simulink model "zynqRadioHWSWQPSKAD9361AD9364SL_UDP_interface"  (R2016a)
settings: Solver=FixedStepDiscrete  SolverMode=SingleTasking  StartTime=0.0  StopTime=inf  RelTol=1e-3
PreLoadFcn:
  | % Ensure SDR libraries are added to path
  | tempradiodev_ = sdrdev('ZC706 and FMCOMMS2/3/4');
  | tempradiodev_.setupSession();
  | clear tempradiodev_; % clean up
  | 
  | sdrzQPSKTxFPGA_params = zynqRadioQPSKTxFPGAAD9361AD9364SL_init;
  | sdrzQPSKrxFPGA = zynqRadioQPSKRxFPGAAD9361AD9364SL_init;
  | 
  | % ARM Tx message
  | txtstr = '*Zynq HW/SW Co-design*';
  | 
  | % Length of data set for transmit
  | DataFrameLength = 10000;
InitFcn:
  | sdrzQPSKTxFPGA_params = zynqRadioQPSKTxFPGAAD9361AD9364SL_init;
  | sdrzQPSKrxFPGA = zynqRadioQPSKRxFPGAAD9361AD9364SL_init;
  | 
  | if (numel(txtstr) > 24)
  |   error('txtstr message must be less than 24 characters');
  | end;
undefined symbols (not defined in the file or in its folder): AXI4, F, Lite, msglen, sdr
libraries: commsequence2 x2, dspsigops x2, commrandsrc2 x1, commutil2 x1, axiinterfacelib x1, zynqlib x1
CloseFcn:
  | clear sdrzQPSKrxFPGA txtstr sdrzQPSKTxFPGA_params DataFrameLength;
settings Model: DataTypeOverride=Off  SimulationMode=external  Creator=The MathWorks, Inc.  LastModifiedBy=The MathWorks, Inc.
settings SolverCC: PositivePriorityOrder=on
settings DataIOCC: LimitDataPoints=on  SaveOutput=off  SaveTime=off
settings OptimizationCC: BlockReduction=off  ConditionallyExecuteInputs=off  OptimizeModelRefInitCode=on  LifeSpan=Inf  MaxStackSize=64
settings DebuggingCC: AlgebraicLoopMsg=error  SingleTaskRateTransMsg=error  AllowSymbolicDim=off  StrictBusMsg=ErrorOnBusTreatedAsVector
settings HardwareCC: ProdBitPerPointer=32  ProdLargestAtomicInteger=Long  ProdLargestAtomicFloat=Double  ProdWordSize=32  ProdLongLongMode=on  ProdHWDeviceType=ARM Compatible->ARM Cortex
settings ModelReferenceCC: PropagateSignalLabelsOutOfModel=off
settings RTWCC: SystemTargetFile=ert.tlc  HardwareBoard=Xilinx Zynq Based Radio Board Target  TemplateMakefile=ert_default_tmf  GenerateReport=on  Toolchain=Xilinx Software Development Kit (SDK)  BuildConfiguration=Faster Runs  IncludeHyperlinkInReport=on  LaunchReport=on  GenerateTraceInfo=on  GenerateTraceReport=on  GenerateTraceReportSl=on  GenerateTraceReportSf=on  GenerateTraceReportEml=on
settings CodeAppCC: ForceParamTrailComments=on  IgnoreCustomStorageClasses=off  OperatorAnnotations=on  SimulinkDataObjDesc=on  SFDataObjDesc=on  MATLABFcnDesc=on  InsertBlockDesc=on  MATLABSourceComments=on
settings ERTTargetCC: SupportVariableSizeSignals=on
settings ConfigurationSet: Description=SimMechanics 2G

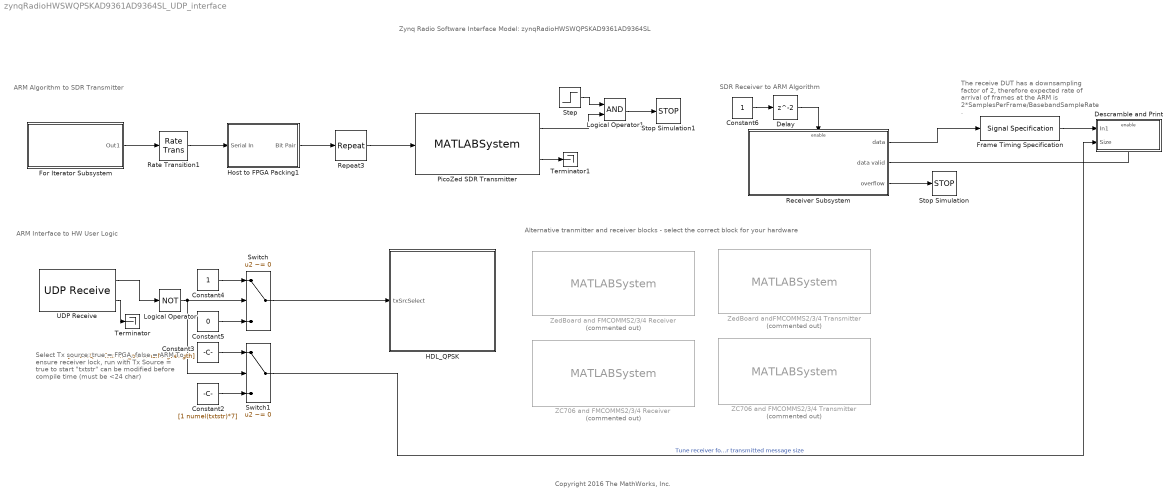
== system zynqRadioHWSWQPSKAD9361AD9364SL_UDP_interface ==
  note: Alternative tranmitter and receiver blocks - select the correct block for your hardware
  note: SDR Receiver to ARM Algorithm
  note: ARM Algorithm to SDR Transmitter
  note: ARM Interface to HW User Logic
  note: Select Tx source:
      | true = FPGA, false = ARM
      |
      | To ensure receiver lock, run with Tx
      | Source = true to start
      |
      | "txtstr" can be modified before
      | compile time (must be <24 char)
  note: Copyright 2016 The MathWorks, Inc.
  note: The receive DUT has a downsampling factor of 2, therefore expected rate of arrival of frames at the ARM is 2*SamplesPerFrame/BasebandSampleRate .
  note: Zynq Radio Software Interface Model: zynqRadioHWSWQPSKAD9361AD9364SL
  Constant2 : Constant  Value=[1 numel(txtstr)*7]  SampleTime=-1
  Constant3 : Constant  Value=[1 sdrzQPSKTxFPGA_params.MsgLength]  SampleTime=-1
  Constant4 : Constant  OutDataTypeStr=boolean  SampleTime=-1
  Constant5 : Constant  Value=0  OutDataTypeStr=boolean  SampleTime=-1
  Constant6 : Constant  SampleTime=2*(DataFrameLength/2)/sdrzQPSKrxFPGA.Fs
  Delay : Delay
  Descramble and Print : Subsystem  TreatAsAtomicUnit=on
  For Iterator Subsystem : Subsystem  TreatAsAtomicUnit=on
  Frame Timing Specification : SignalSpecification  SampleTime=2*(DataFrameLength/2)/sdrzQPSKrxFPGA.Fs
  HDL_QPSK : Subsystem  TreatAsAtomicUnit=on  mask(AXI4-Lite/AXI4 Interface){}
      mask help:
      | This is an automatically generated subsystem block.
      | This contains the AXI interface blocks that communicate with the HDL_QPSK_ip IPCore generated from zynqRadioHWSWQPSKAD9361AD9364SL/HDL_QPSK subsystem.
      mask Display: disp(sprintf('Xilinx Zynq \nAXI Interface'));
  Host to FPGA Packing1 : Subsystem
  Logical Operator : Logic  Operator=NOT  AllPortsSameDT=off  OutDataTypeStr=boolean
  Logical Operator1 : Logic  AllPortsSameDT=off  OutDataTypeStr=boolean
  PicoZed SDR Transmitter : MATLABSystem  Priority=0  InitFcn=sdr.internal.registerBlocks(gcb, 'xpicozedsdr');  System=comm.internal.SDRTxPicoZedSDRSL  IPAddress=192.168.3.2  CenterFrequencySource=Dialog  CenterFrequency=2400000000  GainSource=Dialog  Gain=-10  ChannelMapping=1  BasebandSampleRate=sdrzQPSKrxFPGA.Fs  EnableBurstMode=off  NumFramesInBurst=20  DMATimeoutValue=200e-6  EnableTxPrimingMode=on  blockMode=Codegen  LostSamplesOutputPort=on  OverflowOutputPort=off  DataSourceSelect=Host  DDSFrequency=[ 1000000, 1000000; 1000000, 1000000 ]  DDSPhase=[ 0, 0; 0, 0 ]  DDSScale=[ 250000, 250000; 250000, 250000 ]  BypassUserLogic=off  ShowAdvancedProperties=on  ShowInternalProperties=off  subDeviceList=zynqTransmitter  sdrExecutionMode=HW  dataUDPPort=-1  ctrlUDPPort=-1  FIRCoefficientSize=[ 128; 128 ]  FIRCoefficients=[ 111, -87, 147, -127, -18, -286, -312, -555, -601, -722, -642, -555, -303, -66, 221, 393, 488, 403, 219, -74, -343, -550, -582, -450, -146, 221, 569, 759, 735, 463, 20, -487, -885, -1048, -883, -418, 243, 897, 1340, 1394, 1002, 228, -715, -1549, -1980, -1819, -1028, 217, 1583, 2635, 2980, 2377, 853, -1275, -3435, -4926, -5080, -3454, 40, 5065, 10903, 16581, 21085, 23573, 23573, 21085, 16581, 10903, 5065, 40, -3454, -5080, -4926, -3435, -1275, 853, 2377, 2980, 2635, 1583, 217, -1028, -1819, -1980, -1549, -715, 228, 1002, 1394, 1340, 897, 243, -418, -883, -1048, -885, -487, 20, 463, 735, 759, 569, 221, -146, -450, -582, -550, -343, -74, 219, 403, 488, 393, 221, -66, -303, -555, -642, -722, -601, -555, -312, -286, -18, -127, 147, -87, 111; 382, -200, 711, -41, 645, 36, 346, -194, -119, -543, -472, -646, -404, -312, 45, 197, 413, 346, 241, -93, -373, -680, -755, -689, -356, 51, 515, 795, 870, 609, 136, -488, -1009, -1303, -1191, -712, 69, 885, 1516, 1692, 1336, 468, -662, -1740, -2378, -2329, -1494, -55, 1620, 2995, 3584, 3045, 1368, -1121, -3755, -5708, -6156, -4542, -710, 4969, 11669, 18243, 23486, 26391, 26391, 23486, 18243, 11669, 4969, -710, -4542, -6156, -5708, -3755, -1121, 1368, 3045, 3584, 2995, 1620, -55, -1494, -2329, -2378, -1740, -662, 468, 1336, 1692, 1516, 885, 69, -712, -1191, -1303, -1009, -488, 136, 609, 870, 795, 515, 51, -356, -689, -755, -680, -373, -93, 241, 346, 413, 197, 45, -312, -404, -646, -472, -543, -119, -194, 346, 36, 645, -41, 711, -200, 382 ]  FIRGain=[ 0; -12 ]  FIRDecimInterpFactor=[ 4; 4 ]  AnalogFilterCutoff=[ 2560000; 2560000 ]  FilterPathRates=[ 737280000, 184320000, 61440000, 30720000, 15360000, 3840000; 737280000, 184320000, 61440000, 30720000, 15360000, 3840000 ]  FilterDesignTypeForTx=DefaultFilter  FilterDesignTypeForRx=DefaultFilterFromOther  SimulateUsing=Interpreted execution
      mask Type: comm.internal.SDRTxPicoZedSDRSL
      mask Display:
      | disp(['PicoZed SDR' char(10) 'ARM-FPGA Interface']);
      | port_label('input',1,'data');
      | port_label('output',1,'underflow');
      | port_label('output',2,'overflow');
  Rate Transition1 : RateTransition  OutPortSampleTime=sdrzQPSKTxFPGA_params.FrameTime*(DataFrameLength/(sdrzQPSKTxFPGA_params.DataLength + 2*sdrzQPSKTxFPGA_params.BarkerLength))
  Receiver Subsystem : Subsystem
  Repeat3 : dspsigops/Repeat  N=4  InputProcessing=Columns as channels (frame based)  RateOptions=Allow multirate processing  ic=0  mode=Unused parameter value
  Step : Step  Time=10*DataFrameLength/sdrzQPSKrxFPGA.Fs  SampleTime=DataFrameLength/sdrzQPSKrxFPGA.Fs
  Stop Simulation : Stop
  Stop Simulation1 : Stop
  Switch : Switch  Criteria=u2 ~= 0
  Switch1 : Switch  Criteria=u2 ~= 0
  Terminator : Terminator
  Terminator1 : Terminator
  UDP Receive : zynqlib/UDP Receive  localURL='0.0.0.0'  localPort=25000  remoteURL='0.0.0.0'  remotePort=-1  recvBufferSize=8192  dims=1  signalDatatype=boolean  isVarSize=off  showBlockingTime=on  blockingTime=0  sampletime=2*(DataFrameLength/2)/sdrzQPSKrxFPGA.Fs  blockPlatform=ZYNQ
  ZC706 and FMCOMMS2/3/4 Receiver : MATLABSystem  Priority=0  Commented=on  InitFcn=sdr.internal.registerBlocks(gcb, 'xzc706afmc3');  System=comm.internal.SDRRxZC706FMC234SL  IPAddress=192.168.3.2  CenterFrequencySource=Dialog  CenterFrequency=2400000000  GainSource=AGC Slow Attack  Gain=1  ChannelMapping=1  BasebandSampleRate=sdrzQPSKrxFPGA.Fs  EnableBurstMode=off  NumFramesInBurst=20  OutputDataType=int16  SamplesPerFrame=DataFrameLength/2  LostSamplesOutputPort=on  RSSIOutputPort=off  DMATimeoutValue=200e-6  blockMode=Codegen  EnableQuadratureTracking=on  EnableRFDCTracking=on  EnableBasebandDCTracking=on  BypassUserLogic=off  ShowAdvancedProperties=on  ShowInternalProperties=off  subDeviceList=zynqReceiver  sdrExecutionMode=HW  dataUDPPort=-1  ctrlUDPPort=-1  SourceSelect=RF data  SourceConfiguration1=1023  FIRCoefficientSize=[128;128]  FIRCoefficients=[55 -54 42 -126 -123 -317 -399 -581 -646 -711 -634 -507 -263 -10 255 424 492 401 201 -84 -352 -540 -566 -423 -126 234 562 738 701 429 -5 -490 -866 -1007 -834 -372 266 891 1301 1334 936 178 -733 -1524 -1917 -1731 -944 274 1590 2585 2881 2255 741 -1344 -3435 -4850 -4942 -3285 197 5169 10923 16509 20932 23375 23375 20932 16509 10923 5169 197 -3285 -4942 -4850 -3435 -1344 741 2255 2881 2585 1590 274 -944 -1731 -1917 -1524 -733 178 936 1334 1301 891 266 -372 -834 -1007 -866 -490 -5 429 701 738 562 234 -126 -423 -566 -540 -352 -84 201 401 492 424 255 -10 -263 -507 -634 -711 -646 -581 -399 -317 -123 -126 42 -54 55;190 -88 329 -40 239 -99 -24 -349 -377 -611 -573 -604 -395 -229 66 239 394 350 227 -46 -300 -534 -593 -506 -221 137 512 737 765 526 103 -420 -852 -1069 -947 -512 156 841 1341 1450 1100 333 -638 -1531 -2028 -1922 -1152 115 1544 2677 3099 2535 997 -1205 -3479 -5095 -5345 -3750 -199 4965 11002 16895 21580 24172 24172 21580 16895 11002 4965 -199 -3750 -5345 -5095 -3479 -1205 997 2535 3099 2677 1544 115 -1152 -1922 -2028 -1531 -638 333 1100 1450 1341 841 156 -512 -947 -1069 -852 -420 103 526 765 737 512 137 -221 -506 -593 -534 -300 -46 227 350 394 239 66 -229 -395 -604 -573 -611 -377 -349 -24 -99 239 -40 329 -88 190]  FIRGain=[0;-12]  FIRDecimInterpFactor=[4;4]  AnalogFilterCutoff=[3152524;3161715]  FilterPathRates=[983040000 122880000 61440000 30720000 15360000 3840000;983040000 122880000 61440000 30720000 15360000 3840000]  FilterDesignTypeForTx=DefaultFilterFromOther  FilterDesignTypeForRx=DefaultFilter  BISTLoopbackConfig=No Loopback  BISTPRBSMode=PRBS Disable  BISTToneMode=Tone Disable  BISTToneFrequency=F/32  BISTToneLevel=-6  BISTChannelMask=0  DataIsComplex=on  SimulateUsing=Interpreted execution
      mask Type: comm.internal.SDRRxZC706FMC234SL
      mask Display:
      | disp(['ZC706 and FMCOMMS2/3/4' char(10) 'ARM-FPGA Interface']);
      | port_label('output',1,'data');
      | port_label('output',2,'data valid');
      | port_label('output',3,'overflow');
  ZC706 and FMCOMMS2/3/4 Transmitter : MATLABSystem  Commented=on  InitFcn=sdr.internal.registerBlocks(gcb, 'xzc706afmc3');  System=comm.internal.SDRTxZC706FMC234SL  IPAddress=192.168.3.2  CenterFrequencySource=Dialog  CenterFrequency=2400000000  GainSource=Dialog  Gain=-10  ChannelMapping=1  BasebandSampleRate=sdrzQPSKrxFPGA.Fs  EnableBurstMode=off  NumFramesInBurst=20  DMATimeoutValue=200e-6  EnableTxPrimingMode=on  blockMode=Codegen  LostSamplesOutputPort=on  OverflowOutputPort=off  DataSourceSelect=Host  DDSFrequency=1000000*ones([2 2])  DDSPhase=[0 0;0 0]  DDSScale=250000*ones([2 2])  BypassUserLogic=off  ShowAdvancedProperties=on  ShowInternalProperties=off  subDeviceList=zynqTransmitter  sdrExecutionMode=HW  dataUDPPort=-1  ctrlUDPPort=-1  FIRCoefficientSize=[128;128]  FIRCoefficients=[55 -54 42 -126 -123 -317 -399 -581 -646 -711 -634 -507 -263 -10 255 424 492 401 201 -84 -352 -540 -566 -423 -126 234 562 738 701 429 -5 -490 -866 -1007 -834 -372 266 891 1301 1334 936 178 -733 -1524 -1917 -1731 -944 274 1590 2585 2881 2255 741 -1344 -3435 -4850 -4942 -3285 197 5169 10923 16509 20932 23375 23375 20932 16509 10923 5169 197 -3285 -4942 -4850 -3435 -1344 741 2255 2881 2585 1590 274 -944 -1731 -1917 -1524 -733 178 936 1334 1301 891 266 -372 -834 -1007 -866 -490 -5 429 701 738 562 234 -126 -423 -566 -540 -352 -84 201 401 492 424 255 -10 -263 -507 -634 -711 -646 -581 -399 -317 -123 -126 42 -54 55;190 -88 329 -40 239 -99 -24 -349 -377 -611 -573 -604 -395 -229 66 239 394 350 227 -46 -300 -534 -593 -506 -221 137 512 737 765 526 103 -420 -852 -1069 -947 -512 156 841 1341 1450 1100 333 -638 -1531 -2028 -1922 -1152 115 1544 2677 3099 2535 997 -1205 -3479 -5095 -5345 -3750 -199 4965 11002 16895 21580 24172 24172 21580 16895 11002 4965 -199 -3750 -5345 -5095 -3479 -1205 997 2535 3099 2677 1544 115 -1152 -1922 -2028 -1531 -638 333 1100 1450 1341 841 156 -512 -947 -1069 -852 -420 103 526 765 737 512 137 -221 -506 -593 -534 -300 -46 227 350 394 239 66 -229 -395 -604 -573 -611 -377 -349 -24 -99 239 -40 329 -88 190]  FIRGain=[0;-12]  FIRDecimInterpFactor=[4;4]  AnalogFilterCutoff=[3152524;3161715]  FilterPathRates=[983040000 122880000 61440000 30720000 15360000 3840000;983040000 122880000 61440000 30720000 15360000 3840000]  FilterDesignTypeForTx=DefaultFilter  FilterDesignTypeForRx=DefaultFilterFromOther  SimulateUsing=Interpreted execution
      mask Type: comm.internal.SDRTxZC706FMC234SL
      mask Display:
      | disp(['ZC706 and FMCOMMS2/3/4' char(10) 'ARM-FPGA Interface']);
      | port_label('input',1,'data');
      | port_label('output',1,'underflow');
      | port_label('output',2,'overflow');
  ZedBoard and FMCOMMS2/3/4 Receiver : MATLABSystem  Priority=0  Commented=on  InitFcn=sdr.internal.registerBlocks(gcb, 'xzedboardafmc3');  System=comm.internal.SDRRxZedBoardFMC234SL  IPAddress=192.168.3.2  CenterFrequencySource=Dialog  CenterFrequency=2400000000  GainSource=AGC Slow Attack  Gain=1  ChannelMapping=1  BasebandSampleRate=sdrzQPSKrxFPGA.Fs  EnableBurstMode=off  NumFramesInBurst=20  OutputDataType=int16  SamplesPerFrame=DataFrameLength/2  LostSamplesOutputPort=on  RSSIOutputPort=off  DMATimeoutValue=200e-6  blockMode=Codegen  EnableQuadratureTracking=on  EnableRFDCTracking=on  EnableBasebandDCTracking=on  BypassUserLogic=off  ShowAdvancedProperties=on  ShowInternalProperties=off  subDeviceList=zynqReceiver  sdrExecutionMode=HW  dataUDPPort=-1  ctrlUDPPort=-1  SourceSelect=RF data  SourceConfiguration1=1023  FIRCoefficientSize=[ 128; 128 ]  FIRCoefficients=[ 111, -87, 147, -127, -18, -286, -312, -555, -601, -722, -642, -555, -303, -66, 221, 393, 488, 403, 219, -74, -343, -550, -582, -450, -146, 221, 569, 759, 735, 463, 20, -487, -885, -1048, -883, -418, 243, 897, 1340, 1394, 1002, 228, -715, -1549, -1980, -1819, -1028, 217, 1583, 2635, 2980, 2377, 853, -1275, -3435, -4926, -5080, -3454, 40, 5065, 10903, 16581, 21085, 23573, 23573, 21085, 16581, 10903, 5065, 40, -3454, -5080, -4926, -3435, -1275, 853, 2377, 2980, 2635, 1583, 217, -1028, -1819, -1980, -1549, -715, 228, 1002, 1394, 1340, 897, 243, -418, -883, -1048, -885, -487, 20, 463, 735, 759, 569, 221, -146, -450, -582, -550, -343, -74, 219, 403, 488, 393, 221, -66, -303, -555, -642, -722, -601, -555, -312, -286, -18, -127, 147, -87, 111; 382, -200, 711, -41, 645, 36, 346, -194, -119, -543, -472, -646, -404, -312, 45, 197, 413, 346, 241, -93, -373, -680, -755, -689, -356, 51, 515, 795, 870, 609, 136, -488, -1009, -1303, -1191, -712, 69, 885, 1516, 1692, 1336, 468, -662, -1740, -2378, -2329, -1494, -55, 1620, 2995, 3584, 3045, 1368, -1121, -3755, -5708, -6156, -4542, -710, 4969, 11669, 18243, 23486, 26391, 26391, 23486, 18243, 11669, 4969, -710, -4542, -6156, -5708, -3755, -1121, 1368, 3045, 3584, 2995, 1620, -55, -1494, -2329, -2378, -1740, -662, 468, 1336, 1692, 1516, 885, 69, -712, -1191, -1303, -1009, -488, 136, 609, 870, 795, 515, 51, -356, -689, -755, -680, -373, -93, 241, 346, 413, 197, 45, -312, -404, -646, -472, -543, -119, -194, 346, 36, 645, -41, 711, -200, 382 ]  FIRGain=[ 0; -12 ]  FIRDecimInterpFactor=[ 4; 4 ]  AnalogFilterCutoff=[ 2560000; 2560000 ]  FilterPathRates=[ 737280000, 184320000, 61440000, 30720000, 15360000, 3840000; 737280000, 184320000, 61440000, 30720000, 15360000, 3840000 ]  FilterDesignTypeForTx=DefaultFilterFromOther  FilterDesignTypeForRx=DefaultFilter  BISTLoopbackConfig=No Loopback  BISTPRBSMode=PRBS Disable  BISTToneMode=Tone Disable  BISTToneFrequency=F/32  BISTToneLevel=-6  BISTChannelMask=0  DataIsComplex=on  SimulateUsing=Interpreted execution
      mask Type: comm.internal.SDRRxZedBoardFMC234SL
      mask Display:
      | disp(['ZedBoard and FMCOMMS2/3/4' char(10) 'ARM-FPGA Interface']);
      | port_label('output',1,'data');
      | port_label('output',2,'data valid');
      | port_label('output',3,'overflow');
  ZedBoard andFMCOMMS2/3/4 Transmitter : MATLABSystem  Commented=on  InitFcn=sdr.internal.registerBlocks(gcb, 'xzedboardafmc3');  System=comm.internal.SDRTxZedBoardFMC234SL  IPAddress=192.168.3.2  CenterFrequencySource=Dialog  CenterFrequency=2400000000  GainSource=Dialog  Gain=-10  ChannelMapping=1  BasebandSampleRate=sdrzQPSKrxFPGA.Fs  EnableBurstMode=off  NumFramesInBurst=20  DMATimeoutValue=200e-6  EnableTxPrimingMode=on  blockMode=Codegen  LostSamplesOutputPort=on  OverflowOutputPort=off  DataSourceSelect=Host  DDSFrequency=[ 1000000, 1000000; 1000000, 1000000 ]  DDSPhase=[ 0, 0; 0, 0 ]  DDSScale=[ 250000, 250000; 250000, 250000 ]  BypassUserLogic=off  ShowAdvancedProperties=on  ShowInternalProperties=off  subDeviceList=zynqTransmitter  sdrExecutionMode=HW  dataUDPPort=-1  ctrlUDPPort=-1  FIRCoefficientSize=[ 128; 128 ]  FIRCoefficients=[ 111, -87, 147, -127, -18, -286, -312, -555, -601, -722, -642, -555, -303, -66, 221, 393, 488, 403, 219, -74, -343, -550, -582, -450, -146, 221, 569, 759, 735, 463, 20, -487, -885, -1048, -883, -418, 243, 897, 1340, 1394, 1002, 228, -715, -1549, -1980, -1819, -1028, 217, 1583, 2635, 2980, 2377, 853, -1275, -3435, -4926, -5080, -3454, 40, 5065, 10903, 16581, 21085, 23573, 23573, 21085, 16581, 10903, 5065, 40, -3454, -5080, -4926, -3435, -1275, 853, 2377, 2980, 2635, 1583, 217, -1028, -1819, -1980, -1549, -715, 228, 1002, 1394, 1340, 897, 243, -418, -883, -1048, -885, -487, 20, 463, 735, 759, 569, 221, -146, -450, -582, -550, -343, -74, 219, 403, 488, 393, 221, -66, -303, -555, -642, -722, -601, -555, -312, -286, -18, -127, 147, -87, 111; 382, -200, 711, -41, 645, 36, 346, -194, -119, -543, -472, -646, -404, -312, 45, 197, 413, 346, 241, -93, -373, -680, -755, -689, -356, 51, 515, 795, 870, 609, 136, -488, -1009, -1303, -1191, -712, 69, 885, 1516, 1692, 1336, 468, -662, -1740, -2378, -2329, -1494, -55, 1620, 2995, 3584, 3045, 1368, -1121, -3755, -5708, -6156, -4542, -710, 4969, 11669, 18243, 23486, 26391, 26391, 23486, 18243, 11669, 4969, -710, -4542, -6156, -5708, -3755, -1121, 1368, 3045, 3584, 2995, 1620, -55, -1494, -2329, -2378, -1740, -662, 468, 1336, 1692, 1516, 885, 69, -712, -1191, -1303, -1009, -488, 136, 609, 870, 795, 515, 51, -356, -689, -755, -680, -373, -93, 241, 346, 413, 197, 45, -312, -404, -646, -472, -543, -119, -194, 346, 36, 645, -41, 711, -200, 382 ]  FIRGain=[ 0; -12 ]  FIRDecimInterpFactor=[ 4; 4 ]  AnalogFilterCutoff=[ 2560000; 2560000 ]  FilterPathRates=[ 737280000, 184320000, 61440000, 30720000, 15360000, 3840000; 737280000, 184320000, 61440000, 30720000, 15360000, 3840000 ]  FilterDesignTypeForTx=DefaultFilter  FilterDesignTypeForRx=DefaultFilterFromOther  SimulateUsing=Interpreted execution
      mask Type: comm.internal.SDRTxZedBoardFMC234SL
      mask Display:
      | disp(['ZedBoard and FMCOMMS2/3/4' char(10) 'ARM-FPGA Interface']);
      | port_label('input',1,'data');
      | port_label('output',1,'underflow');
      | port_label('output',2,'overflow');
  wires:
  Repeat3/1 -> PicoZed SDR Transmitter/1
  Frame Timing Specification/1 -> Descramble and Print/1(In1)
  Switch/1 -> HDL_QPSK/1(txSrcSelect)
  Constant4/1 -> Switch/1
  Constant5/1 -> Switch/3
  Constant2/1 -> Switch1/3
  Constant3/1 -> Switch1/1
  Switch1/1 -> Descramble and Print/2(Size)  "Tune receiver for transmitted message size"
  PicoZed SDR Transmitter/2 -> Terminator1/1
  For Iterator Subsystem/1(Out1) -> Rate Transition1/1
  Host to FPGA Packing1/1(Bit Pair) -> Repeat3/1
  Rate Transition1/1 -> Host to FPGA Packing1/1(Serial In)
  Receiver Subsystem/1(data) -> Frame Timing Specification/1
  Receiver Subsystem/2(data valid) -> Descramble and Print/Enable
  Receiver Subsystem/3(overflow) -> Stop Simulation/1
  Constant6/1 -> Delay/1
  Delay/1 -> Receiver Subsystem/Enable
  Logical Operator/1 -> Switch1/2, Switch/2
  UDP Receive/1 -> Logical Operator/1
  Step/1 -> Logical Operator1/1
  PicoZed SDR Transmitter/1 -> Logical Operator1/2
  UDP Receive/2 -> Terminator/1
  Logical Operator1/1 -> Stop Simulation1/1

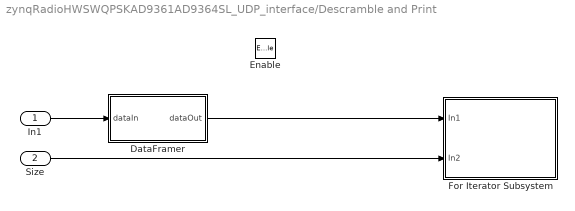
== system zynqRadioHWSWQPSKAD9361AD9364SL_UDP_interface/Descramble and Print ==
  In1 : Inport
  Size : Inport  Port=2
  Enable : EnablePort  PropagateVarSize=During execution
  DataFramer : MATLAB Function  TreatAsAtomicUnit=on
  For Iterator Subsystem : Subsystem  TreatAsAtomicUnit=on
  wires:
  In1/1 -> DataFramer/1(dataIn)
  DataFramer/1(dataOut) -> For Iterator Subsystem/1(In1)
  Size/1 -> For Iterator Subsystem/2(In2)

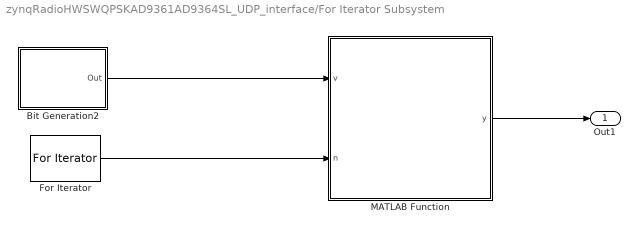
== system zynqRadioHWSWQPSKAD9361AD9364SL_UDP_interface/For Iterator Subsystem ==
  Bit Generation2 : Subsystem
      mask Display: disp('Bits Generation')
  For Iterator : ForIterator  IterationLimit=(DataFrameLength/(sdrzQPSKTxFPGA_params.DataLength + 2*sdrzQPSKTxFPGA_params.BarkerLength))-1  IndexMode=Zero-based
  MATLAB Function : MATLAB Function  TreatAsAtomicUnit=on
  Out1 : Outport
  wires:
  MATLAB Function/1(y) -> Out1/1
  For Iterator/1 -> MATLAB Function/2(n)
  Bit Generation2/1(Out) -> MATLAB Function/1(v)

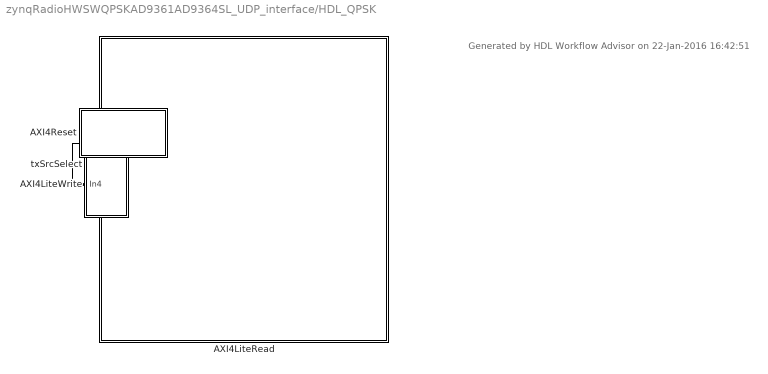
== system zynqRadioHWSWQPSKAD9361AD9364SL_UDP_interface/HDL_QPSK ==
  note: Generated by HDL Workflow Advisor on 22-Jan-2016 16:42:51
  txSrcSelect : Inport
  AXI4LiteRead : Subsystem  Priority=10
  AXI4LiteWrite : Subsystem  Priority=1
  AXI4Reset : Subsystem  mask(System Initialize){ShowInLibBrowser=0}
      mask prompts: ShowInLibBrowser "Simulink:masks:CustCodeMaskParam1_MP"
      settings: CopyFcn=cccopyfcn(gcb)  OpenFcn=ccopenfcn('System Initialize Function')
      mask Help: eval('feval(''rtwprivate'',''rtwhelpview'',''rtw_sys_initialize_block'')');
      mask Display: disp('System\nInitialize');
  wires:
  txSrcSelect/1 -> AXI4LiteWrite/1(In4)

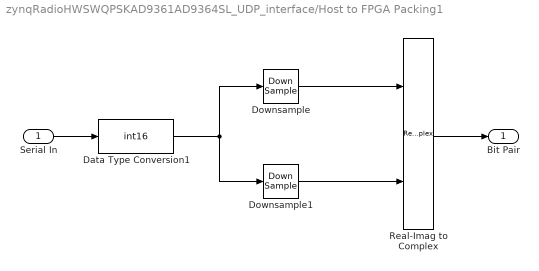
== system zynqRadioHWSWQPSKAD9361AD9364SL_UDP_interface/Host to FPGA Packing1 ==
  Serial In : Inport
  Data Type Conversion1 : DataTypeConversion  OutDataTypeStr=int16
  Downsample : DownSample  RateOptions=Allow multirate processing
  Downsample1 : DownSample  phase=1  RateOptions=Allow multirate processing
  Real-Imag to Complex : RealImagToComplex
  Bit Pair : Outport
  wires:
  Downsample/1 -> Real-Imag to Complex/1
  Serial In/1 -> Data Type Conversion1/1
  Data Type Conversion1/1 -> Downsample1/1, Downsample/1
  Downsample1/1 -> Real-Imag to Complex/2
  Real-Imag to Complex/1 -> Bit Pair/1

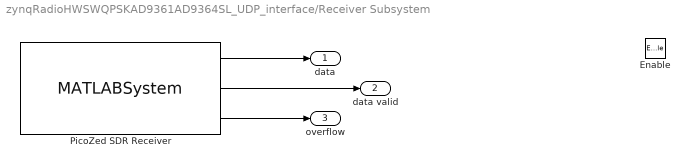
== system zynqRadioHWSWQPSKAD9361AD9364SL_UDP_interface/Receiver Subsystem ==
  Enable : EnablePort
  PicoZed SDR Receiver : MATLABSystem  InitFcn=sdr.internal.registerBlocks(gcb, 'xpicozedsdr');  System=comm.internal.SDRRxPicoZedSDRSL  IPAddress=192.168.3.2  CenterFrequencySource=Dialog  CenterFrequency=2400000000  GainSource=AGC Fast Attack  Gain=1  ChannelMapping=1  BasebandSampleRate=sdrzQPSKrxFPGA.Fs  EnableBurstMode=off  NumFramesInBurst=20  OutputDataType=int16  SamplesPerFrame=DataFrameLength/2  LostSamplesOutputPort=on  RSSIOutputPort=off  DMATimeoutValue=200e-6  blockMode=Codegen  EnableQuadratureTracking=on  EnableRFDCTracking=on  EnableBasebandDCTracking=on  BypassUserLogic=off  ShowAdvancedProperties=on  ShowInternalProperties=off  subDeviceList=zynqReceiver  sdrExecutionMode=HW  dataUDPPort=-1  ctrlUDPPort=-1  SourceSelect=RF data  SourceConfiguration1=1023  FIRCoefficientSize=[ 128; 128 ]  FIRCoefficients=[ 111, -87, 147, -127, -18, -286, -312, -555, -601, -722, -642, -555, -303, -66, 221, 393, 488, 403, 219, -74, -343, -550, -582, -450, -146, 221, 569, 759, 735, 463, 20, -487, -885, -1048, -883, -418, 243, 897, 1340, 1394, 1002, 228, -715, -1549, -1980, -1819, -1028, 217, 1583, 2635, 2980, 2377, 853, -1275, -3435, -4926, -5080, -3454, 40, 5065, 10903, 16581, 21085, 23573, 23573, 21085, 16581, 10903, 5065, 40, -3454, -5080, -4926, -3435, -1275, 853, 2377, 2980, 2635, 1583, 217, -1028, -1819, -1980, -1549, -715, 228, 1002, 1394, 1340, 897, 243, -418, -883, -1048, -885, -487, 20, 463, 735, 759, 569, 221, -146, -450, -582, -550, -343, -74, 219, 403, 488, 393, 221, -66, -303, -555, -642, -722, -601, -555, -312, -286, -18, -127, 147, -87, 111; 382, -200, 711, -41, 645, 36, 346, -194, -119, -543, -472, -646, -404, -312, 45, 197, 413, 346, 241, -93, -373, -680, -755, -689, -356, 51, 515, 795, 870, 609, 136, -488, -1009, -1303, -1191, -712, 69, 885, 1516, 1692, 1336, 468, -662, -1740, -2378, -2329, -1494, -55, 1620, 2995, 3584, 3045, 1368, -1121, -3755, -5708, -6156, -4542, -710, 4969, 11669, 18243, 23486, 26391, 26391, 23486, 18243, 11669, 4969, -710, -4542, -6156, -5708, -3755, -1121, 1368, 3045, 3584, 2995, 1620, -55, -1494, -2329, -2378, -1740, -662, 468, 1336, 1692, 1516, 885, 69, -712, -1191, -1303, -1009, -488, 136, 609, 870, 795, 515, 51, -356, -689, -755, -680, -373, -93, 241, 346, 413, 197, 45, -312, -404, -646, -472, -543, -119, -194, 346, 36, 645, -41, 711, -200, 382 ]  FIRGain=[ 0; -12 ]  FIRDecimInterpFactor=[ 4; 4 ]  AnalogFilterCutoff=[ 2560000; 2560000 ]  FilterPathRates=[ 737280000, 184320000, 61440000, 30720000, 15360000, 3840000; 737280000, 184320000, 61440000, 30720000, 15360000, 3840000 ]  FilterDesignTypeForTx=DefaultFilterFromOther  FilterDesignTypeForRx=DefaultFilter  BISTLoopbackConfig=No Loopback  BISTPRBSMode=PRBS Disable  BISTToneMode=Tone Disable  BISTToneFrequency=F/32  BISTToneLevel=-6  BISTChannelMask=0  DataIsComplex=on  SimulateUsing=Interpreted execution
      mask Type: comm.internal.SDRRxPicoZedSDRSL
      mask Display:
      | disp(['PicoZed SDR' char(10) 'ARM-FPGA Interface']);
      | port_label('output',1,'data');
      | port_label('output',2,'data valid');
      | port_label('output',3,'overflow');
  data : Outport
  data valid : Outport  Port=2
  overflow : Outport  Port=3
  wires:
  PicoZed SDR Receiver/2 -> data valid/1
  PicoZed SDR Receiver/1 -> data/1
  PicoZed SDR Receiver/3 -> overflow/1

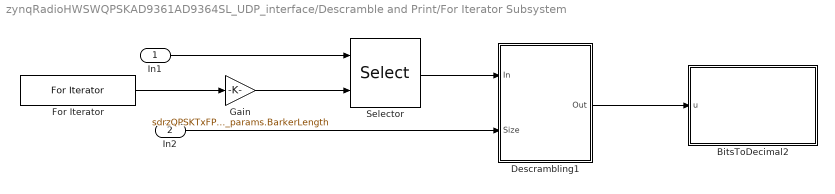
== system zynqRadioHWSWQPSKAD9361AD9364SL_UDP_interface/Descramble and Print/For Iterator Subsystem ==
  In1 : Inport
  In2 : Inport  Port=2
  BitsToDecimal2 : MATLAB Function  TreatAsAtomicUnit=on
  Descrambling1 : Subsystem
      mask Display: disp('Descrambling')
  For Iterator : ForIterator  IterationLimit=(DataFrameLength/(sdrzQPSKTxFPGA_params.DataLength + 2*sdrzQPSKTxFPGA_params.BarkerLength))-1  IndexMode=Zero-based
  Gain : Gain  Gain=sdrzQPSKTxFPGA_params.DataLength + 2*sdrzQPSKTxFPGA_params.BarkerLength  OutDataTypeStr=int32
  Selector : Selector  IndexMode=Zero-based  IndexOptions=Starting index (port)  Indices=[sdrzQPSKrxFPGA.BarkerLength*log2(sdrzQPSKrxFPGA.M)+1:sdrzQPSKrxFPGA.FrameSize*log2(sdrzQPSKrxFPGA.M)]  OutputSizes=sdrzQPSKTxFPGA_params.DataLength + 2*sdrzQPSKTxFPGA_params.BarkerLength
  wires:
  Descrambling1/1(Out) -> BitsToDecimal2/1(u)
  In2/1 -> Descrambling1/2(Size)
  In1/1 -> Selector/1
  Selector/1 -> Descrambling1/1(In)
  Gain/1 -> Selector/2
  For Iterator/1 -> Gain/1

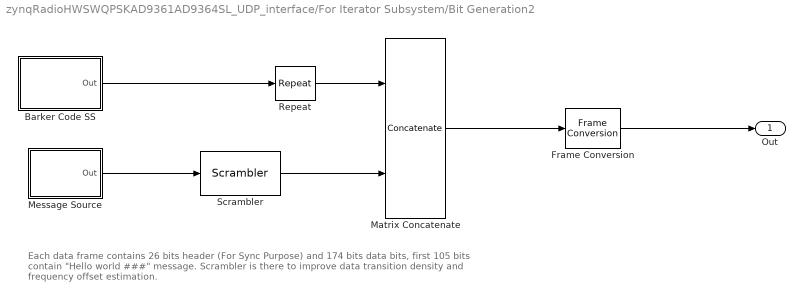
== system zynqRadioHWSWQPSKAD9361AD9364SL_UDP_interface/For Iterator Subsystem/Bit Generation2 ==
  note: Each data frame contains 26 bits header (For Sync Purpose) and 174 bits data bits,
      | first 105 bits contain "Hello world ###" message. Scrambler is there to improve data
      | transition density and frequency offset estimation.
  Barker Code SS : Subsystem
      mask Display: disp('Unipolar\nBarker Code')
  Frame Conversion : FrameConversion  InheritSamplingMode=off  OutFrame=Sample-based
  Matrix Concatenate : Concatenate  Mode=Multidimensional array
  Message Source : Subsystem
      mask Display: disp('Message\nSource')
  Repeat : dspsigops/Repeat  N=2  InputProcessing=Columns as channels (frame based)  RateOptions=Enforce single-rate processing  ic=0  mode=Unused parameter value
  Scrambler : commsequence2/Scrambler  M=2  poly=[1 1 1 0 1]  iniStaSource=Dialog Parameter  ini_sta=[0 0 0 0]  resetViaPort=off
  Out : Outport
  wires:
  Frame Conversion/1 -> Out/1
  Matrix Concatenate/1 -> Frame Conversion/1
  Barker Code SS/1(Out) -> Repeat/1
  Repeat/1 -> Matrix Concatenate/1
  Scrambler/1 -> Matrix Concatenate/2
  Message Source/1(Out) -> Scrambler/1

== system zynqRadioHWSWQPSKAD9361AD9364SL_UDP_interface/HDL_QPSK/AXI4LiteRead ==

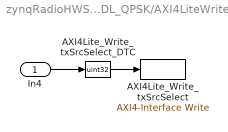
== system zynqRadioHWSWQPSKAD9361AD9364SL_UDP_interface/HDL_QPSK/AXI4LiteWrite ==
  In4 : Inport
  AXI4Lite_Write_txSrcSelect : axiinterfacelib/AXI4-Interface Write  Priority=7  AXIInterfaceType=AXI4-Lite  DeviceName=/dev/mwipcore1  RegisterOffset=hex2dec('100')  blockPlatform=ZYNQ  SimulateUsing=Interpreted execution
  AXI4Lite_Write_txSrcSelect_DTC : DataTypeConversion  OutDataTypeStr=uint32  ConvertRealWorld=Stored Integer (SI)
  wires:
  In4/1 -> AXI4Lite_Write_txSrcSelect_DTC/1
  AXI4Lite_Write_txSrcSelect_DTC/1 -> AXI4Lite_Write_txSrcSelect/1

== system zynqRadioHWSWQPSKAD9361AD9364SL_UDP_interface/HDL_QPSK/AXI4Reset ==

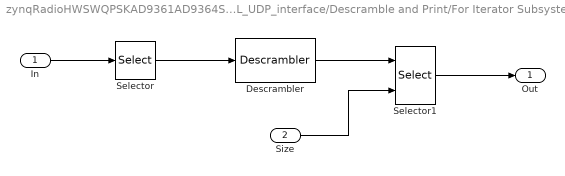
== system zynqRadioHWSWQPSKAD9361AD9364SL_UDP_interface/Descramble and Print/For Iterator Subsystem/Descrambling1 ==
  In : Inport
  Size : Inport  Port=2
  Descrambler : commsequence2/Descrambler  M=2  poly=[1 1 1 0 1]  iniStaSource=Dialog Parameter  ini_sta=[0 0 0 0]  resetViaPort=off
  Selector : Selector  IndexOptions=Index vector (dialog)  Indices=[sdrzQPSKrxFPGA.BarkerLength*log2(sdrzQPSKrxFPGA.M)+1:sdrzQPSKrxFPGA.FrameSize*log2(sdrzQPSKrxFPGA.M)]  OutputSizes=1
  Selector1 : Selector  IndexOptions=Starting and ending indices (port)  Indices=[1:msglen]  OutputSizes=1
  Out : Outport
  wires:
  Selector/1 -> Descrambler/1
  In/1 -> Selector/1
  Selector1/1 -> Out/1
  Descrambler/1 -> Selector1/1
  Size/1 -> Selector1/2

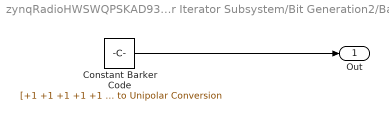
== system zynqRadioHWSWQPSKAD9361AD9364SL_UDP_interface/For Iterator Subsystem/Bit Generation2/Barker Code SS ==
  Constant Barker Code : Constant  Value=|  VectorParams1D=off  OutDataTypeStr=double  SampleTime=-1
      | [+1 +1 +1 +1 +1 -1 -1 +1 +1 -1 +1 -1 +1
      | ].' > 0  % Bipolar to Unipolar Conversion
  Out : Outport
  wires:
  Constant Barker Code/1 -> Out/1

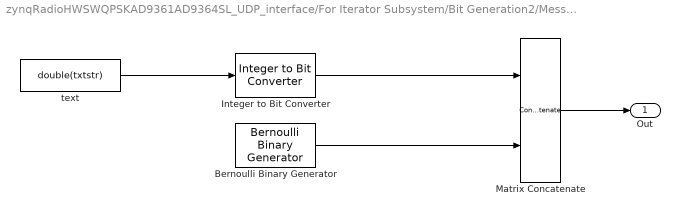
== system zynqRadioHWSWQPSKAD9361AD9364SL_UDP_interface/For Iterator Subsystem/Bit Generation2/Message Source ==
  Bernoulli Binary Generator : commrandsrc2/Bernoulli Binary Generator  P=0.5  seed=61  Ts=-1  frameBased=on  sampPerFrame=sdrzQPSKTxFPGA_params.DataLength - numel(txtstr)*7  orient=off  outDataType=double
  Integer to Bit Converter : commutil2/Integer to Bit Converter  nbits=7  signedInputValues=Unsigned  bitOrder=MSB first  outDtype=Inherit via internal rule
  Matrix Concatenate : Concatenate  Mode=Multidimensional array
  text : Constant  Value=double(txtstr)  SampleTime=-1
  Out : Outport
  wires:
  text/1 -> Integer to Bit Converter/1
  Integer to Bit Converter/1 -> Matrix Concatenate/1
  Matrix Concatenate/1 -> Out/1
  Bernoulli Binary Generator/1 -> Matrix Concatenate/2

== matlab function zynqRadioHWSWQPSKAD9361AD9364SL_UDP_interface/Descramble and Print/For Iterator Subsystem/BitsToDecimal2 ==
  data: u input
function BitsToASCII(u)
%#codegen
% Convert bits to ASCII message.
% Convert binary-valued column vector to 7-bit decimal values.
w = [64 32 16 8 4 2 1]; % binary digit weighting
Nbits = numel(u);
Ny = Nbits/7;
y = zeros(1,Ny);
for i = 0:Ny-1
    y(i+1) = w*u(7*i+(1:7));
end

% replace the non-printable characters with "^" char(94) 
% to indicate an error 
y(y > 126)= 94; 
y(y < 32) = 94;
% Display ASCII message to command window
fprintf('%s\n',char(y));

== matlab function zynqRadioHWSWQPSKAD9361AD9364SL_UDP_interface/For Iterator Subsystem/MATLAB Function ==
  data: y output; v input; n input
function y = fcn(v,n)
%#codegen
persistent output;

% Length of generated data set, this must match the DataFrameLength
% associated with the rest of the model
DataFrameLength = 10000;

% Message length (sdrzQPSKTxFPGA_params.DataLength + 2*sdrzQPSKTxFPGA_params.BarkerLength)
MessageLength = 200;

if isempty(output)
    output = zeros(DataFrameLength,1);
end
startIdx = n*MessageLength+1;
endIdx = startIdx+MessageLength;
output(startIdx:endIdx,1) = v;
y = output;

== matlab function zynqRadioHWSWQPSKAD9361AD9364SL_UDP_interface/Descramble and Print/DataFramer ==
  data: dataIn input; dataOut output
function dataOut = fcn(dataIn)
%#codegen


nData = 2*numel(dataIn);

b1 = real(dataIn);
b2 = imag(dataIn);

dataOut = logical(reshape([b1,b2]',nData,1));
